simulink model "closeloop"  (R2019b)
settings: Solver=VariableStepAuto  StartTime=0.0  StopTime=10.0  RelTol=1e-3
values from neighbouring files (symbols this model uses):
  Ksim = SelectedController    [NLPAR.m]    (also in NOMINAL_CONTROLLER.m = Knom; RESULTS.m; WORST.m)
undefined symbols (not defined in the file or in its folder): segway
settings Model: Creator=Abolfazl  LastModifiedBy=Abolfazl

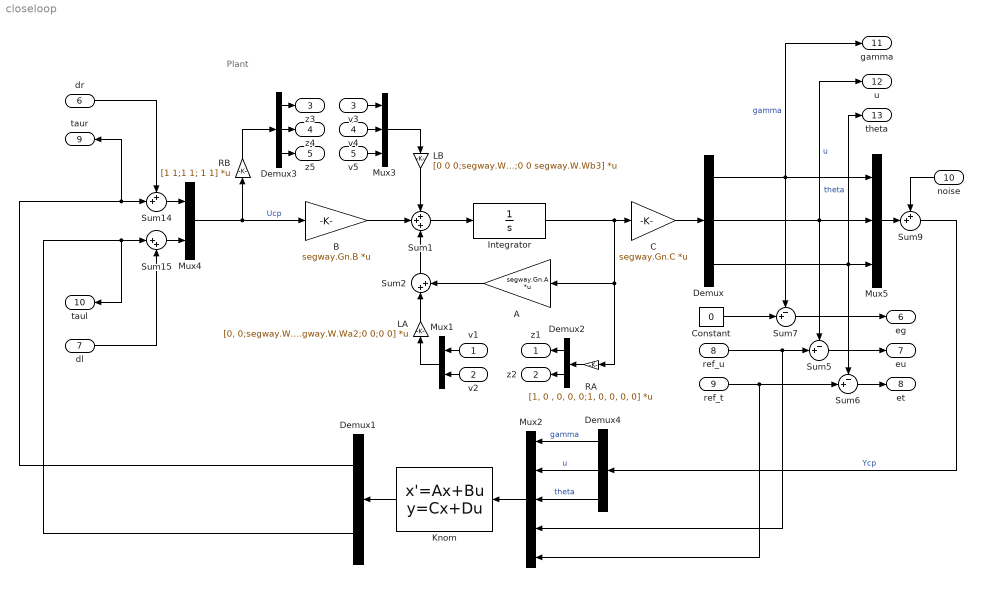
== system closeloop ==
  note: Plant
  v1 : Inport
  v2 : Inport  Port=2
  v3 : Inport  Port=3
  v4 : Inport  Port=4
  v5 : Inport  Port=5
  dr : Inport  Port=6
  dl : Inport  Port=7
  ref_u : Inport  Port=8
  ref_t : Inport  Port=9
  noise : Inport  Port=10
  A : Gain  Gain=segway.Gn.A  Multiplication=Matrix(K*u)
  B : Gain  Gain=segway.Gn.B  Multiplication=Matrix(K*u)
  C : Gain  Gain=segway.Gn.C  Multiplication=Matrix(K*u)
  Constant : Constant  Value=0
  Demux : Demux  Outputs=3
  Demux1 : Demux  Outputs=2
  Demux2 : Demux  Outputs=2
  Demux3 : Demux  Outputs=3
  Demux4 : Demux  Outputs=3
  Integrator : Integrator
  Knom : StateSpace  A=Ksim.A  B=Ksim.B  C=Ksim.C  D=Ksim.D  InitialCondition=0
  LA : Gain  Gain=[0, 0;segway.W.Wa1 0;0 segway.W.Wa2;0 0;0 0]  Multiplication=Matrix(K*u)
  LB : Gain  Gain=[0 0 0;segway.W.Wb1 0 0;0 segway.W.Wb2 0;0 0 0;0 0 segway.W.Wb3]  Multiplication=Matrix(K*u)
  Mux1 : Mux  Inputs=2
  Mux2 : Mux  Inputs=5
  Mux3 : Mux  Inputs=3
  Mux4 : Mux  Inputs=2
  Mux5 : Mux  Inputs=3
  RA : Gain  Gain=[1, 0 , 0, 0, 0;1, 0, 0, 0, 0]  Multiplication=Matrix(K*u)
  RB : Gain  Gain=[1 1;1 1; 1 1]  Multiplication=Matrix(K*u)
  Sum1 : Sum  Inputs=+++
  Sum14 : Sum  Inputs=++|
  Sum15 : Sum  Inputs=|++
  Sum2 : Sum  Inputs=|++
  Sum5 : Sum  Inputs=-+|
  Sum6 : Sum  Inputs=-+|
  Sum7 : Sum  Inputs=-+|
  Sum9 : Sum  Inputs=++|
  z1 : Outport
  z2 : Outport  Port=2
  z3 : Outport  Port=3
  z4 : Outport  Port=4
  z5 : Outport  Port=5
  eg : Outport  Port=6
  eu : Outport  Port=7
  et : Outport  Port=8
  taur : Outport  Port=9
  taul : Outport  Port=10
  gamma : Outport  Port=11
  u : Outport  Port=12
  theta : Outport  Port=13
  wires:
  Mux2/1 -> Knom/1
  Knom/1 -> Demux1/1
  Demux1/1 -> Sum14/2, taur/1
  Demux/3 -> theta/1, Mux5/3, Sum6/1  "theta"
  Demux2/1 -> z1/1
  Sum5/1 -> eu/1
  Demux1/2 -> taul/1, Sum15/1
  Mux1/1 -> LA/1
  LA/1 -> Sum2/1
  Sum2/1 -> Sum1/3
  v4/1 -> Mux3/2
  v3/1 -> Mux3/1
  Mux4/1 -> RB/1, B/1  "Ucp"
  A/1 -> Sum2/2
  Demux3/3 -> z5/1
  RB/1 -> Demux3/1
  Demux2/2 -> z2/1
  B/1 -> Sum1/2
  ref_u/1 -> Mux2/4, Sum5/2
  Sum6/1 -> et/1
  dl/1 -> Sum15/2
  v1/1 -> Mux1/1
  dr/1 -> Sum14/1
  RA/1 -> Demux2/1
  LB/1 -> Sum1/1
  Sum1/1 -> Integrator/1
  Mux3/1 -> LB/1
  Integrator/1 -> C/1, A/1, RA/1
  v2/1 -> Mux1/2
  v5/1 -> Mux3/3
  Demux3/1 -> z3/1
  Demux/1 -> gamma/1, Mux5/1, Sum7/1  "gamma"
  Demux3/2 -> z4/1
  Sum14/1 -> Mux4/1
  ref_t/1 -> Mux2/5, Sum6/2
  Demux/2 -> u/1, Mux5/2, Sum5/1  "u"
  Sum15/1 -> Mux4/2
  Constant/1 -> Sum7/2
  Sum7/1 -> eg/1
  C/1 -> Demux/1
  Mux5/1 -> Sum9/2
  Sum9/1 -> Demux4/1  "Ycp"
  Demux4/2 -> Mux2/2  "u"
  Demux4/1 -> Mux2/1  "gamma"
  Demux4/3 -> Mux2/3  "theta"
  noise/1 -> Sum9/1
